simulink model "respnose_sim"  (R2025b)
settings: Solver=VariableStepAuto  StartTime=0.0  StopTime=10.0  RelTol=1e-3
settings Model: Creator=iwa  LastModifiedBy=iwa

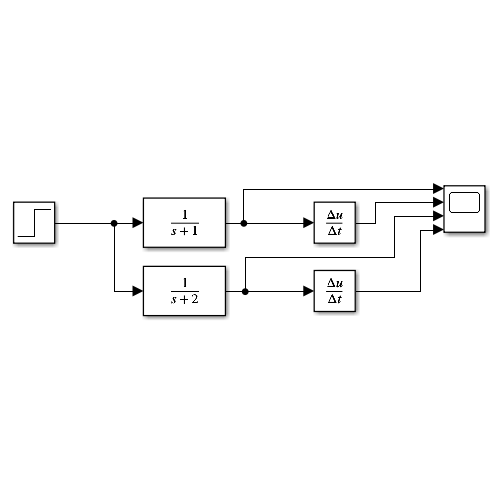
[thumbnail: Simulink's stored preview of the top-level diagram]
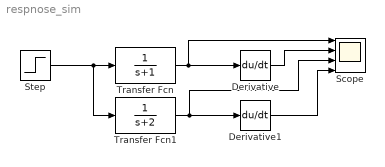
== system respnose_sim ==
  Derivative : Derivative
  Derivative1 : Derivative
  Scope : Scope  NumInputPorts=4
      settings: ActiveDisplayYMinimum=-0.12499999999999908  ActiveDisplayYMaximum=1.124999999999992
  Step : Step  SampleTime=0
  Transfer Fcn : TransferFcn  Denominator=[1 1]
  Transfer Fcn1 : TransferFcn  Denominator=[1 2]
  wires:
  Step/1 -> Transfer Fcn1/1, Transfer Fcn/1
  Transfer Fcn/1 -> Scope/1, Derivative/1
  Derivative/1 -> Scope/2
  Transfer Fcn1/1 -> Scope/3, Derivative1/1
  Derivative1/1 -> Scope/4
